simulink model "Vehicle"  (R2018a)
settings: Solver=VariableStepAuto  StartTime=0.0  StopTime=10.0  RelTol=1e-3
values from neighbouring files (symbols this model uses):
  lr = 1.6    [SimVehicle.m]    (also in Untitled.m)
  m = 1575    [SimVehicle.m]    (also in Untitled.m)
  yaw0_ego = 0    [SimVehicle.m]    (also in Untitled.m)
libraries: autolibshared x1
settings Model: Creator=jdrjk  LastModifiedBy=jdrjk
settings DataIOCC: SaveFinalState=on  SaveCompleteFinalSimState=on  SaveState=on

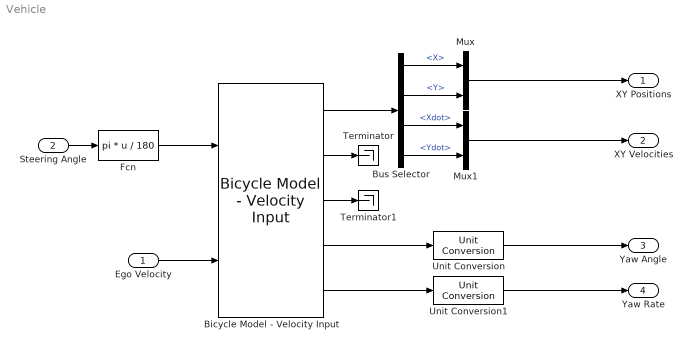
== system Vehicle ==
  Ego Velocity : Inport
  Steering Angle : Inport  Port=2
  Bicycle Model - Velocity Input : autolibshared/Bicycle Model - Velocity Input  trackMode=Single (bicycle)  inputMode=External longitudinal forces  frontSteerMode=on  rearSteerMode=off  windMode=off  muMode=off  extFMode=off  extMMode=off  aMode=3  NF=2  NR=2  m=m  a=lf  b=lr  h=0.35  X_o=x0_ego  xdot_o=0  CalphaMode=off  sigmaMode=on  w=[1.4,1.4]  Cy_f=Cf  Cy_r=Cr  sigma_f=.1  sigma_r=.1  alpha_f_brk=[-.1 .1]  Cy_f_data=[-9e3 9e3]  alpha_r_brk=[-.1 .1]  Cy_r_data=[-9e3 9e3]  Y_o=y0_ego  ydot_o=0  Izz=Iz  psi_o=yaw0_ego*pi/180  r_o=0  Af=2  Cd=.3  Cl=.1  Cpm=.1  beta_w=[0:0.01:0.3]  Cs=[0:0.03:0.9]  Cym=[0:0.01:0.3]  Pabs=101325  Tair=273  g=9.81  mu=1  xdot_tol=.01  Fznom=5000  Fxtire_sat=1e6  Fytire_sat=1e6
      settings: SourceProductName=Powertrain Blockset  SourceProductBaseCode=PW
  Bus Selector : BusSelector  OutputSignals=InertFrm.FrntAxl.Disp.X,InertFrm.FrntAxl.Disp.Y,InertFrm.FrntAxl.Vel.Xdot,InertFrm.FrntAxl.Vel.Ydot
  Fcn : Fcn  Expr=pi * u / 180
  Mux : Mux  Inputs=2
  Mux1 : Mux  Inputs=2
  Terminator : Terminator
  Terminator1 : Terminator
  Unit Conversion : UnitConversion  OutputType=Inherit: Inherit via back propagation
  Unit Conversion1 : UnitConversion  OutputType=Inherit: Inherit via back propagation
  XY Positions : Outport  Unit=m
  XY Velocities : Outport  Port=2  Unit=m/s
  Yaw Angle : Outport  Port=3  Unit=deg
  Yaw Rate : Outport  Port=4  Unit=degree/s
  wires:
  Bus Selector/4 -> Mux1/2  "<Ydot>"
  Ego Velocity/1 -> Bicycle Model - Velocity Input/2
  Bicycle Model - Velocity Input/3 -> Terminator1/1
  Bicycle Model - Velocity Input/2 -> Terminator/1
  Bus Selector/1 -> Mux/1  "<X>"
  Mux/1 -> XY Positions/1
  Bus Selector/3 -> Mux1/1  "<Xdot>"
  Unit Conversion/1 -> Yaw Angle/1
  Bicycle Model - Velocity Input/5 -> Unit Conversion1/1
  Bicycle Model - Velocity Input/1 -> Bus Selector/1
  Unit Conversion1/1 -> Yaw Rate/1
  Fcn/1 -> Bicycle Model - Velocity Input/1
  Bicycle Model - Velocity Input/4 -> Unit Conversion/1
  Bus Selector/2 -> Mux/2  "<Y>"
  Mux1/1 -> XY Velocities/1
  Steering Angle/1 -> Fcn/1
